simulink model "s_3d_crane_jib_pos_cntrl"  (Simulink 6.6)
settings: Solver=FixedStepDiscrete  StartTime=0.0  StopTime=15  FixedStep=0.001  RelTol=1e-3
values from neighbouring files (symbols this model uses):
  A_J = A    [setup_3d_crane.m]
  B_J = B    [setup_3d_crane.m]
  C_J = C    [setup_3d_crane.m]
  D_J = D    [setup_3d_crane.m]
  IMAX_AMP = 7    [setup_3d_crane.m]
  K_J = lqr(A_J,B_J,Q_J,R_J)    [setup_3d_crane.m]
  wf_gamma = 2 * pi * 2.0    (= 12.5663706144)    [setup_3d_crane.m]
  wf_x = 2 * pi * 50    (= 314.159265359)    [setup_3d_crane.m]
undefined symbols (not defined in the file or in its folder): DiscIntNeverNeededParam, qc_get_step_size
libraries: quarc_library x6, simulink x3, simulink_extras x1
settings Model: Creator=MLevis  LastModifiedBy=MLevis  ExtModeTrigDuration=10000
settings SolverCC: PositivePriorityOrder=on
settings RTWCC: SystemTargetFile=quarc_windows.tlc  TemplateMakefile=quarc_default_tmf  Description=QuaRC Win32 Target  ProcessScript=quarc_windows_make_rtw_hook
settings STFCustomTargetCC: TargetFcnLib=ansi_tfl_tmw.mat  TargetPreCompLibLocation=C:\DOCUME~1\ALLUSE~1\APPLIC~1\QuaRC\lib\2007a\windows\release  GenFloatMathFcnCalls=ANSI_C  SystemTargetFile=quarc_windows.tlc
settings GRTTargetCC: TargetPreCompLibLocation=C:\DOCUME~1\ALLUSE~1\APPLIC~1\QuaRC\lib\2007a\windows\release  MatFileLogging=off  ExtMode=on  ExtModeMexFile=quarc_comm

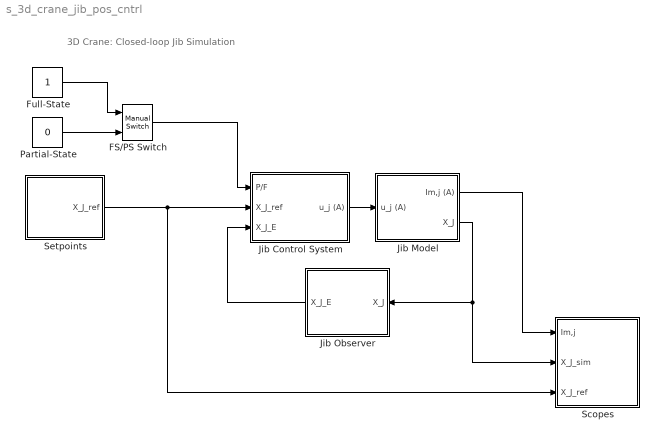
== system s_3d_crane_jib_pos_cntrl ==
  note: 3D Crane: Closed-loop Jib Simulation
  FS/PS Switch : simulink/Signal Routing/Manual Switch  SystemSampleTime=-1  sw=1  action=0  varsize=off
  Full-State : Constant
  Jib Control System : Subsystem
  Jib Model : Subsystem
  Jib Observer : Subsystem  Orientation=left
  Partial-State : Constant  Value=0
  Scopes : Subsystem
  Setpoints : Subsystem
  wires:
  Jib Control System/1(u_j (A)) -> Jib Model/1(u_j (A))
  Setpoints/1(X_J_ref) -> Scopes/3(X_J_ref), Jib Control System/2(X_J_ref)
  Full-State/1 -> FS/PS Switch/1
  Partial-State/1 -> FS/PS Switch/2
  FS/PS Switch/1 -> Jib Control System/1(P/F)
  Jib Model/1(Im,j (A)) -> Scopes/1(Im,j)
  Jib Model/2(X_J) -> Scopes/2(X_J_sim), Jib Observer/1(X_J)
  Jib Observer/1(X_J_E) -> Jib Control System/3(X_J_E)

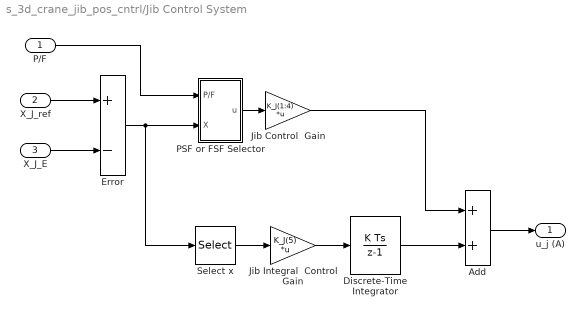
== system s_3d_crane_jib_pos_cntrl/Jib Control System ==
  P/F : Inport
  X_J_ref : Inport  Port=2
  X_J_E : Inport  Port=3
  Add : Sum  OutScaling=2^-10
  Discrete-Time Integrator : DiscreteIntegrator  SampleTime=qc_get_step_size  LimitOutput=on  UpperSaturationLimit=2  LowerSaturationLimit=-2  ICPrevOutput=DiscIntNeverNeededParam  ICPrevScaledInput=DiscIntNeverNeededParam
  Error : Sum  Inputs=+-  OutScaling=2^-10
  Jib Control  Gain : Gain  Gain=K_J(1:4)  Multiplication=Matrix(K*u)
  Jib Integral  Control Gain : Gain  Gain=K_J(5)  Multiplication=Matrix(K*u)
  PSF or FSF Selector : Subsystem
  Select x : Selector  IndexOptions=Index vector (dialog)  Indices=1  OutputSizes=1  InputPortWidth=4
  u_j (A) : Outport
  wires:
  PSF or FSF Selector/1(u) -> Jib Control  Gain/1
  P/F/1 -> PSF or FSF Selector/1(P/F)
  Add/1 -> u_j (A)/1
  Discrete-Time Integrator/1 -> Add/2
  Jib Control  Gain/1 -> Add/1
  Jib Integral  Control Gain/1 -> Discrete-Time Integrator/1
  Select x/1 -> Jib Integral  Control Gain/1
  X_J_E/1 -> Error/2
  X_J_ref/1 -> Error/1
  Error/1 -> PSF or FSF Selector/2(X), Select x/1

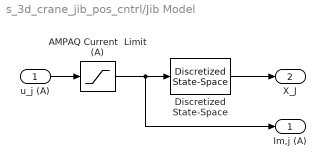
== system s_3d_crane_jib_pos_cntrl/Jib Model ==
  u_j (A) : Inport
  AMPAQ Current  Limit (A) : Saturate  UpperLimit=IMAX_AMP  LowerLimit=-IMAX_AMP
  Discretized State-Space : quarc_library/Discrete/Discretized State-Space  SystemSampleTime=-1  A=[A_J(1:4,1:4)]  B=[B_J(1:4)]  C=[C_J]  D=[D_J]  x0=[0]  method=tustin  Ts=qc_get_step_size
  Im,j (A) : Outport
  X_J : Outport  Port=2
  wires:
  Discretized State-Space/1 -> X_J/1
  AMPAQ Current  Limit (A)/1 -> Im,j (A)/1, Discretized State-Space/1
  u_j (A)/1 -> AMPAQ Current  Limit (A)/1

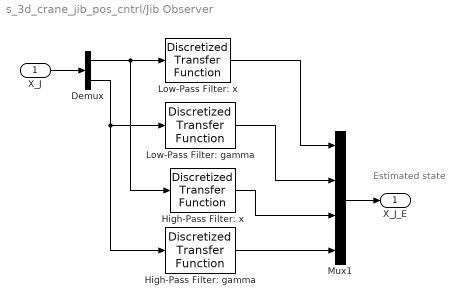
== system s_3d_crane_jib_pos_cntrl/Jib Observer ==
  note: Estimated state
  X_J : Inport
  Demux : Demux  Outputs=2
  High-Pass Filter: gamma : quarc_library/Discrete/Discretized Transfer Function  SystemSampleTime=-1  num=[wf_gamma 0]  den=[1 wf_gamma]  method=tustin  Ts=qc_get_step_size
  High-Pass Filter: x : quarc_library/Discrete/Discretized Transfer Function  SystemSampleTime=-1  num=[wf_x 0]  den=[1 wf_x]  method=tustin  Ts=qc_get_step_size
  Low-Pass Filter: gamma : quarc_library/Discrete/Discretized Transfer Function  SystemSampleTime=-1  num=[wf_gamma]  den=[1 wf_gamma]  method=tustin  Ts=qc_get_step_size
  Low-Pass Filter: x : quarc_library/Discrete/Discretized Transfer Function  SystemSampleTime=-1  num=[wf_x]  den=[1 wf_x]  method=tustin  Ts=qc_get_step_size
  Mux1 : Mux
  X_J_E : Outport
  wires:
  X_J/1 -> Demux/1
  High-Pass Filter: gamma/1 -> Mux1/4
  High-Pass Filter: x/1 -> Mux1/3
  Mux1/1 -> X_J_E/1
  Low-Pass Filter: x/1 -> Mux1/1
  Low-Pass Filter: gamma/1 -> Mux1/2
  Demux/1 -> Low-Pass Filter: x/1, High-Pass Filter: x/1
  Demux/2 -> Low-Pass Filter: gamma/1, High-Pass Filter: gamma/1

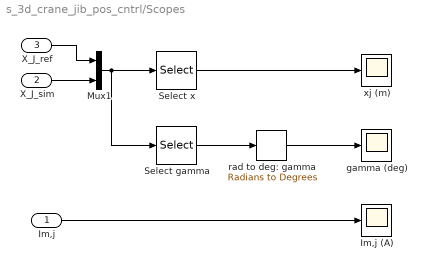
== system s_3d_crane_jib_pos_cntrl/Scopes ==
  Im,j : Inport
  X_J_sim : Inport  Port=2
  X_J_ref : Inport  Port=3
  Im,j (A) : Scope
      settings: TimeRange=15  YMin=-1.117279536301703  YMax=1.013399074108925  SaveName=ScopeData3
  Mux1 : Mux  Inputs=2
  Select gamma : Selector  IndexOptions=Index vector (dialog)  Indices=[2 6]  OutputSizes=1  InputPortWidth=6
  Select x : Selector  IndexOptions=Index vector (dialog)  Indices=[1 5]  OutputSizes=1  InputPortWidth=6
  gamma (deg) : Scope
      settings: TimeRange=15  YMin=-30  YMax=30  SaveName=ScopeData9
  rad to deg: gamma : simulink_extras/Transformations/Radians to Degrees  SystemSampleTime=-1
  xj (m) : Scope
      settings: TimeRange=15  YMin=0  YMax=0.6
  wires:
  Im,j/1 -> Im,j (A)/1
  rad to deg: gamma/1 -> gamma (deg)/1
  Select x/1 -> xj (m)/1
  Select gamma/1 -> rad to deg: gamma/1
  X_J_ref/1 -> Mux1/1
  X_J_sim/1 -> Mux1/2
  Mux1/1 -> Select x/1, Select gamma/1

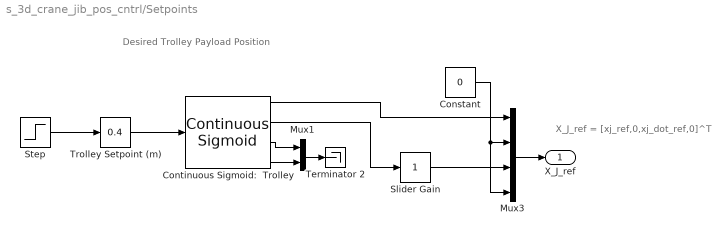
== system s_3d_crane_jib_pos_cntrl/Setpoints ==
  note: X_J_ref = [xj_ref,0,xj_dot_ref,0]^T
  note: Desired Trolley Payload Position
  Constant : Constant  Value=0
  Continuous Sigmoid:  Trolley : quarc_library/Sources/Sigmoids/Continuous Sigmoid  params_source=Internal (dialog parameters)  max_velocity=0.75  max_acceleration=1.5  initial_position=0  initial_velocity=0  hold_off=0.5  input_sample_time=-1  output_sample_time=qc_get_step_size
  Mux1 : Mux  Inputs=2
  Mux3 : Mux
  Slider Gain : simulink/Math Operations/Slider Gain  SystemSampleTime=-1  low=0  gain=1  high=1
  Step : Step  SampleTime=0
  Terminator 2 : Terminator
  Trolley Setpoint (m) : simulink/Math Operations/Slider Gain  SystemSampleTime=-1  low=-0.4  gain=0.4  high=0.4
  X_J_ref : Outport
  wires:
  Slider Gain/1 -> Mux3/3
  Step/1 -> Trolley Setpoint (m)/1
  Mux1/1 -> Terminator 2/1
  Trolley Setpoint (m)/1 -> Continuous Sigmoid:  Trolley/1
  Mux3/1 -> X_J_ref/1
  Continuous Sigmoid:  Trolley/1 -> Mux3/1
  Constant/1 -> Mux3/2, Mux3/4
  Continuous Sigmoid:  Trolley/3 -> Mux1/1
  Continuous Sigmoid:  Trolley/4 -> Mux1/2
  Continuous Sigmoid:  Trolley/2 -> Slider Gain/1

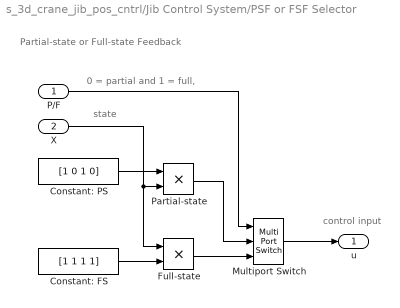
== system s_3d_crane_jib_pos_cntrl/Jib Control System/PSF or FSF Selector ==
  note: control input
  note: state
  note: 0 = partial and 1 = full,
  note: Partial-state or Full-state Feedback
  P/F : Inport
  X : Inport  Port=2
  Constant: FS : Constant  Value=[1 1 1 1]
  Constant: PS : Constant  Value=[1 0 1 0]
  Full-state : Product  RndMeth=Zero
  Multiport Switch : MultiPortSwitch  Inputs=2  zeroidx=on
  Partial-state : Product  RndMeth=Zero
  u : Outport
  wires:
  X/1 -> Full-state/1, Partial-state/2
  P/F/1 -> Multiport Switch/1
  Multiport Switch/1 -> u/1
  Full-state/1 -> Multiport Switch/3
  Partial-state/1 -> Multiport Switch/2
  Constant: PS/1 -> Partial-state/1
  Constant: FS/1 -> Full-state/2
